simulink model "chap17_02_106_mdl"  (R2013b)
settings: Solver=FixedStepDiscrete  SolverMode=SingleTasking  StartTime=0.0  StopTime=10.0  FixedStep=0.1  RelTol=1e-3  SampleTimeConstraint=Specified
settings Model: Creator=Administrator  LastModifiedBy=sunzx.fnst
settings OptimizationCC: OptimizeModelRefInitCode=on  LifeSpan=1
settings RTWCC: SystemTargetFile=ert.tlc  GenCodeOnly=on  TemplateMakefile=ert_default_tmf  Description=Embedded Coder  GenerateReport=on  ProcessScript=ert_make_rtw_hook  IncludeHyperlinkInReport=on  LaunchReport=on
settings CodeAppCC: IgnoreCustomStorageClasses=off
settings ERTTargetCC: CodeReplacementLibrary=ANSI_C  GenerateSampleERTMain=on  ERTCustomFileTemplate=example_file_process.tlc  EnableUserReplacementTypes=on

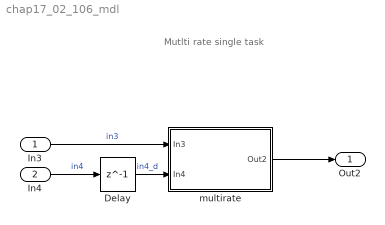
== system chap17_02_106_mdl ==
  note: Mutlti rate single task
  In3 : Inport  OutDataTypeStr=FLOAT32  SampleTime=1
  In4 : Inport  Port=2  OutDataTypeStr=UINT16  SampleTime=2
  Delay : Delay  DelayLength=1  InitialCondition=0  StateName=delay
  multirate : Subsystem  TreatAsAtomicUnit=on
      settings: RTWFcnNameOpts=Use subsystem name
  Out2 : Outport  OutDataTypeStr=boolean
  wires:
  In3/1 -> multirate/1(In3)  "in3"
  In4/1 -> Delay/1  "in4"
  multirate/1(Out2) -> Out2/1
  Delay/1 -> multirate/2(In4)  "in4_d"

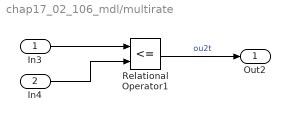
== system chap17_02_106_mdl/multirate ==
  In3 : Inport  OutDataTypeStr=FLOAT32
  In4 : Inport  Port=2  OutDataTypeStr=UINT16
  Relational Operator1 : RelationalOperator  Operator=<=  OutDataTypeStr=boolean
  Out2 : Outport  OutDataTypeStr=boolean
  wires:
  Relational Operator1/1 -> Out2/1  "ou2t"
  In3/1 -> Relational Operator1/1
  In4/1 -> Relational Operator1/2
